simulink model "p1_2022a"  (R2022a)
settings: Solver=VariableStepAuto  StartTime=0.0  StopTime=10.0  RelTol=1e-3
values from neighbouring files (symbols this model uses):
  KD_1st = KP_1st* .5*L    (= 7.50234448265e-08)    [PID_DESING.m]
  KI_1st = KP_1st/(2*L)    (= 0.468896530166)    [PID_DESING.m]
  KP_1st = 1.2*(L/T)    (= 0.000375117224133)    [PID_DESING.m]
  Wn1 = 1/(R1*C1)    (= 0.980392156863)    [scondorder.m]
  Wn2 = 1/(R2*C2)    (= 1.25)    [scondorder.m]
  Wn3 = 1/(R3*C3)    (= 1.11111111111)    [scondorder.m]
  zeta1 = 3*R1*C1/(2*Wn1*(R1^2)*(C1^2))    (= 1.5)    [scondorder.m]
  zeta2 = 3*R2*C2/(2*Wn2*(R2^2)*(C2^2))    (= 1.5)    [scondorder.m]
  zeta3 = 3*R3*C3/(2*Wn3*(R3^2)*(C3^2))    (= 1.5)    [scondorder.m]
undefined symbols (not defined in the file or in its folder): KD1, KD2, KD3, KI1, KI2, KI3, KP1, KP2, KP3
settings Model: Creator=ascom  LastModifiedBy=ascom
settings ModelReferenceCC: EnableRefExpFcnMdlSchedulingChecks=off
settings RTWCC: Description=Generic Real-Time Target

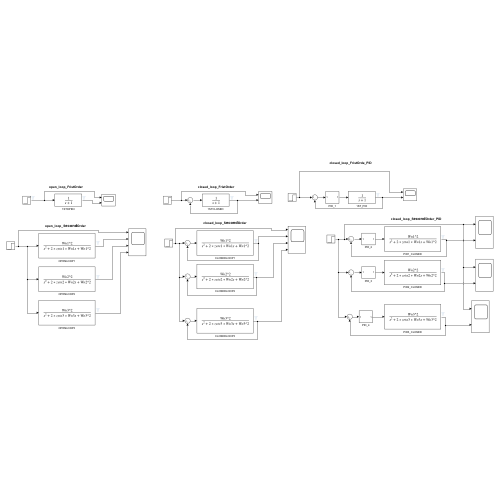
[thumbnail: Simulink's stored preview of the top-level diagram]
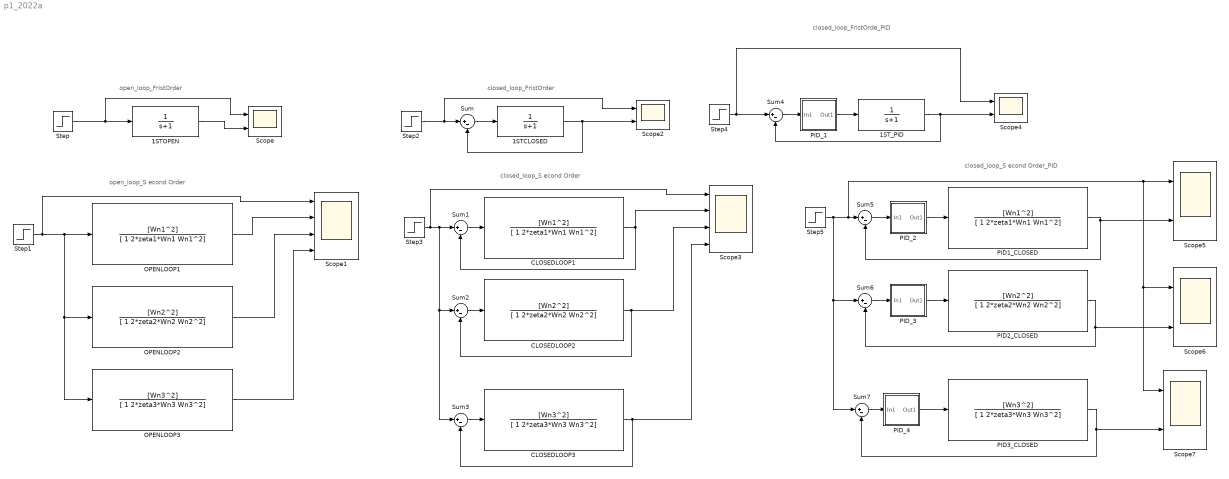
== system p1_2022a ==
  note: closed_loop_FristOrder
  note: open_loop_FristOrder
  note: open_loop_S econd Order
  note: closed_loop_S econd Order
  note: closed_loop_FristOrde_PID
  note: closed_loop_S econd Order_PID
  1STCLOSED : TransferFcn  Denominator=[1 1]
  1STOPEN : TransferFcn  Denominator=[1 1]
  1ST_PID : TransferFcn  Denominator=[1 1]
  CLOSEDLOOP1 : TransferFcn  Numerator=[Wn1^2]  Denominator=[ 1 2*zeta1*Wn1 Wn1^2]
  CLOSEDLOOP2 : TransferFcn  Numerator=[Wn2^2]  Denominator=[ 1 2*zeta2*Wn2 Wn2^2]
  CLOSEDLOOP3 : TransferFcn  Numerator=[Wn3^2]  Denominator=[ 1 2*zeta3*Wn3 Wn3^2]
  OPENLOOP1 : TransferFcn  Numerator=[Wn1^2]  Denominator=[ 1 2*zeta1*Wn1 Wn1^2]
  OPENLOOP2 : TransferFcn  Numerator=[Wn2^2]  Denominator=[ 1 2*zeta2*Wn2 Wn2^2]
  OPENLOOP3 : TransferFcn  Numerator=[Wn3^2]  Denominator=[ 1 2*zeta3*Wn3 Wn3^2]
  PID1_CLOSED : TransferFcn  Numerator=[Wn1^2]  Denominator=[ 1 2*zeta1*Wn1 Wn1^2]
  PID2_CLOSED : TransferFcn  Numerator=[Wn2^2]  Denominator=[ 1 2*zeta2*Wn2 Wn2^2]
  PID3_CLOSED : TransferFcn  Numerator=[Wn3^2]  Denominator=[ 1 2*zeta3*Wn3 Wn3^2]
  PID_1 : Subsystem
  PID_2 : Subsystem
  PID_3 : Subsystem
  PID_4 : Subsystem
  Scope{,2,4..7} (6 alike) : Scope  NumInputPorts=2
  Scope1 : Scope  NumInputPorts=4
  Scope3 : Scope  NumInputPorts=4
  Step{,1..5} (6 alike) : Step  SampleTime=0
  Sum{,1..7} (8 alike) : Sum  Inputs=|+-
  wires:
  Sum2/1 -> CLOSEDLOOP2/1
  Step3/1 -> Scope3/1, Sum1/1, Sum3/1, Sum2/1
  CLOSEDLOOP1/1 -> Sum1/2, Scope3/2
  CLOSEDLOOP2/1 -> Sum2/2, Scope3/3
  Sum1/1 -> CLOSEDLOOP1/1
  CLOSEDLOOP3/1 -> Sum3/2, Scope3/4
  Step2/1 -> Sum/1, Scope2/1
  1STCLOSED/1 -> Scope2/2, Sum/2
  OPENLOOP3/1 -> Scope1/4
  OPENLOOP1/1 -> Scope1/2
  Step1/1 -> Scope1/1, OPENLOOP3/1, OPENLOOP2/1, OPENLOOP1/1
  Step/1 -> Scope/1, 1STOPEN/1
  OPENLOOP2/1 -> Scope1/3
  1STOPEN/1 -> Scope/2
  Sum3/1 -> CLOSEDLOOP3/1
  1ST_PID/1 -> Sum4/2, Scope4/2
  Step4/1 -> Scope4/1, Sum4/1
  PID3_CLOSED/1 -> Scope7/2, Sum7/2
  PID2_CLOSED/1 -> Scope6/2, Sum6/2
  PID1_CLOSED/1 -> Sum5/2, Scope5/2
  Sum/1 -> 1STCLOSED/1
  Step5/1 -> Sum7/1, Sum6/1, Scope7/1, Scope6/1, Scope5/1, Sum5/1
  Sum4/1 -> PID_1/1(In1)
  PID_1/1(Out1) -> 1ST_PID/1
  PID_2/1(Out1) -> PID1_CLOSED/1
  Sum5/1 -> PID_2/1(In1)
  PID_3/1(Out1) -> PID2_CLOSED/1
  Sum6/1 -> PID_3/1(In1)
  Sum7/1 -> PID_4/1(In1)
  PID_4/1(Out1) -> PID3_CLOSED/1

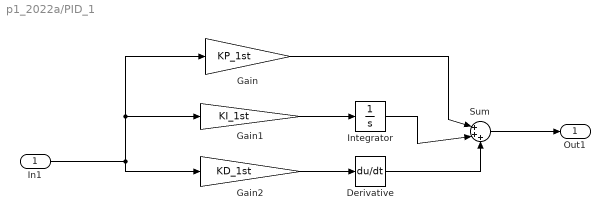
== system p1_2022a/PID_1 ==
  In1 : Inport
  Derivative : Derivative
  Gain : Gain  Gain=KP_1st
  Gain1 : Gain  Gain=KI_1st
  Gain2 : Gain  Gain=KD_1st
  Integrator : Integrator
  Sum : Sum  Inputs=|+++
  Out1 : Outport
  wires:
  Gain1/1 -> Integrator/1
  Gain2/1 -> Derivative/1
  Sum/1 -> Out1/1
  Gain/1 -> Sum/1
  Integrator/1 -> Sum/2
  Derivative/1 -> Sum/3
  In1/1 -> Gain1/1, Gain/1, Gain2/1

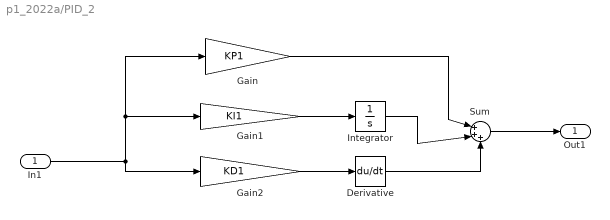
== system p1_2022a/PID_2 ==
  In1 : Inport
  Derivative : Derivative
  Gain : Gain  Gain=KP1
  Gain1 : Gain  Gain=KI1
  Gain2 : Gain  Gain=KD1
  Integrator : Integrator
  Sum : Sum  Inputs=|+++
  Out1 : Outport
  wires:
  In1/1 -> Gain2/1, Gain/1, Gain1/1
  Derivative/1 -> Sum/3
  Integrator/1 -> Sum/2
  Gain/1 -> Sum/1
  Sum/1 -> Out1/1
  Gain2/1 -> Derivative/1
  Gain1/1 -> Integrator/1

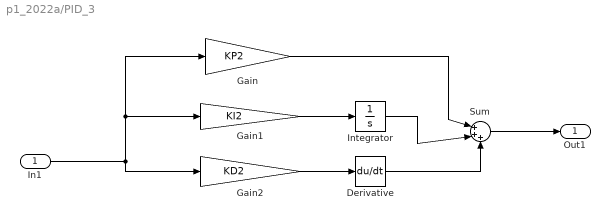
== system p1_2022a/PID_3 ==
  In1 : Inport
  Derivative : Derivative
  Gain : Gain  Gain=KP2
  Gain1 : Gain  Gain=KI2
  Gain2 : Gain  Gain=KD2
  Integrator : Integrator
  Sum : Sum  Inputs=|+++
  Out1 : Outport
  wires:
  Gain1/1 -> Integrator/1
  Gain2/1 -> Derivative/1
  Sum/1 -> Out1/1
  Gain/1 -> Sum/1
  Integrator/1 -> Sum/2
  Derivative/1 -> Sum/3
  In1/1 -> Gain1/1, Gain/1, Gain2/1

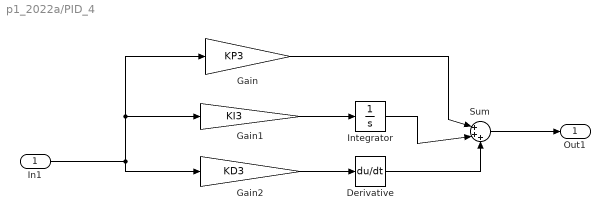
== system p1_2022a/PID_4 ==
  In1 : Inport
  Derivative : Derivative
  Gain : Gain  Gain=KP3
  Gain1 : Gain  Gain=KI3
  Gain2 : Gain  Gain=KD3
  Integrator : Integrator
  Sum : Sum  Inputs=|+++
  Out1 : Outport
  wires:
  In1/1 -> Gain2/1, Gain/1, Gain1/1
  Derivative/1 -> Sum/3
  Integrator/1 -> Sum/2
  Gain/1 -> Sum/1
  Sum/1 -> Out1/1
  Gain2/1 -> Derivative/1
  Gain1/1 -> Integrator/1
